simulink model "Simulacion_b"  (R2021a)
settings: Solver=VariableStepAuto  StartTime=0.0  StopTime=500  RelTol=1e-3
values from neighbouring files (symbols this model uses):
  Qi = 8/(1000*60)    (= 0.000133333333333)    [TP1.m]
  ue = double(ue)    [TP1.m]
  x1e = 0.45    [TP1.m]
  ye = 0.45    [TP1.m]
libraries: cstblocks x3
settings Model: Creator=amddy  LastModifiedBy=Jorge_Sarmiento

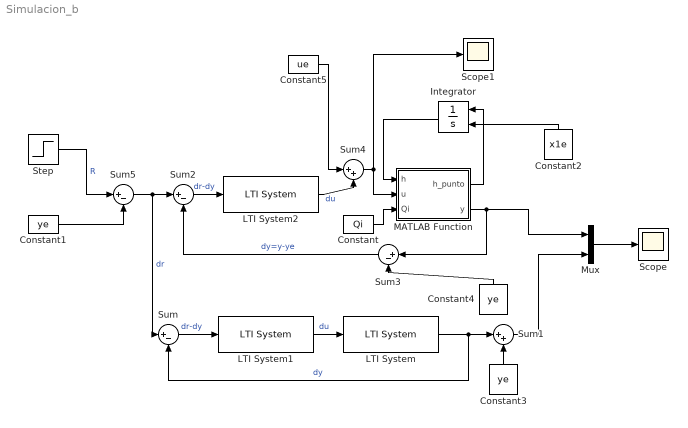
== system Simulacion_b ==
  Constant : Constant  Value=Qi
  Constant1 : Constant  Value=ye
  Constant2 : Constant  Value=x1e
  Constant3 : Constant  Value=ye
  Constant4 : Constant  Value=ye
  Constant5 : Constant  Value=ue
  Integrator : Integrator  InitialConditionSource=external
  LTI System : cstblocks/LTI System  sys=G  IC=[]
  LTI System1 : cstblocks/LTI System  sys=C  IC=[]
  LTI System2 : cstblocks/LTI System  sys=C  IC=[]
  MATLAB Function : MATLAB Function  TreatAsAtomicUnit=on
  Mux : Mux  Inputs=2
  Scope : Scope
  Scope1 : Scope
  Step : Step  Time=0  After=0.55  SampleTime=0
  Sum{,2..3,5} (4 alike) : Sum  Inputs=|+-
  Sum1 : Sum  Inputs=|++
  Sum4 : Sum  Inputs=|++
  wires:
  Integrator/1 -> MATLAB Function/1(h)
  Constant/1 -> MATLAB Function/3(Qi)
  MATLAB Function/1(h_punto) -> Integrator/1
  Mux/1 -> Scope/1
  Constant2/1 -> Integrator/2
  LTI System/1 -> Sum/2, Sum1/1  "dy"
  MATLAB Function/2(y) -> Sum3/1, Mux/1
  Sum1/1 -> Mux/2
  Constant3/1 -> Sum1/2
  Sum/1 -> LTI System1/1  "dr-dy"
  LTI System1/1 -> LTI System/1  "du"
  LTI System2/1 -> Sum4/2  "du"
  Sum2/1 -> LTI System2/1  "dr-dy"
  Sum3/1 -> Sum2/2  "dy=y-ye"
  Constant4/1 -> Sum3/2
  Constant5/1 -> Sum4/1
  Sum4/1 -> MATLAB Function/2(u), Scope1/1
  Sum5/1 -> Sum/1, Sum2/1  "dr"
  Step/1 -> Sum5/1  "R"
  Constant1/1 -> Sum5/2

== matlab function Simulacion_b/MATLAB Function ==
  data: h input; h_punto output; u input; Qi input; y output
function [h_punto,y] = fcn(h,u,Qi)

d_tuberia= 10.65e-3; % metros
lb = 10e-2;  % metros
la= 40e-2; % metros
S= pi*((d_tuberia/2)^2); % metros^2
L=0.9; % metros
g=9.81; % metros/seg^2

h_punto= (Qi - S*u*sqrt(2*g*h))/(lb + (la - lb)*h/L);
y=h;
end
